simulink model "model"  (R2014a)
settings: Solver=ode45  StartTime=0.0  StopTime=10.0  MaxStep=1  MinStep=1  RelTol=1e-3
undefined symbols (not defined in the file or in its folder): a1, a2, a3, b1, b2, b3, H, T
settings Model: Creator=L13-4  LastModifiedBy=L13-4

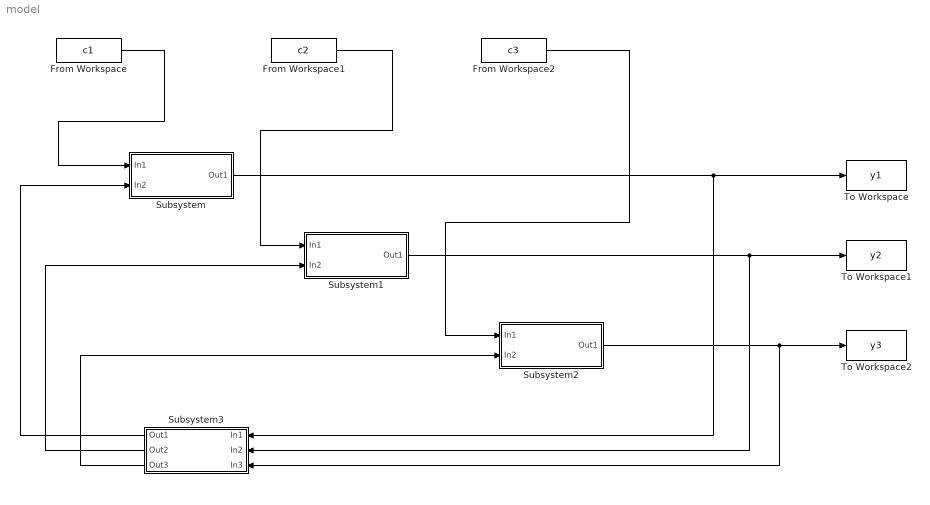
== system model ==
  From Workspace : FromWorkspace  VariableName=c1  SampleTime=0
  From Workspace1 : FromWorkspace  VariableName=c2  SampleTime=0
  From Workspace2 : FromWorkspace  VariableName=c3  SampleTime=0
  Subsystem : Subsystem
  Subsystem1 : Subsystem
  Subsystem2 : Subsystem
  Subsystem3 : Subsystem
  To Workspace : ToWorkspace  VariableName=y1  SampleTime=-1
  To Workspace1 : ToWorkspace  VariableName=y2  SampleTime=-1
  To Workspace2 : ToWorkspace  VariableName=y3  SampleTime=-1
  wires:
  From Workspace/1 -> Subsystem/1(In1)
  Subsystem/1(Out1) -> Subsystem3/1(In1), To Workspace/1
  From Workspace1/1 -> Subsystem1/1(In1)
  From Workspace2/1 -> Subsystem2/1(In1)
  Subsystem1/1(Out1) -> Subsystem3/2(In2), To Workspace1/1
  Subsystem2/1(Out1) -> Subsystem3/3(In3), To Workspace2/1
  Subsystem3/1(Out1) -> Subsystem/2(In2)
  Subsystem3/2(Out2) -> Subsystem1/2(In2)
  Subsystem3/3(Out3) -> Subsystem2/2(In2)

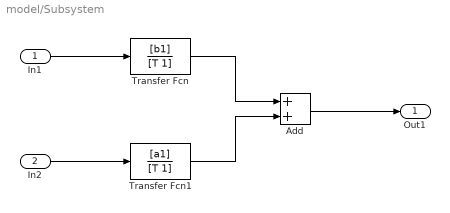
== system model/Subsystem ==
  In1 : Inport
  In2 : Inport  Port=2
  Add : Sum
  Transfer Fcn : TransferFcn  Numerator=[b1]  Denominator=[T 1]
  Transfer Fcn1 : TransferFcn  Numerator=[a1]  Denominator=[T 1]
  Out1 : Outport
  wires:
  In2/1 -> Transfer Fcn1/1
  Transfer Fcn1/1 -> Add/2
  Add/1 -> Out1/1
  Transfer Fcn/1 -> Add/1
  In1/1 -> Transfer Fcn/1

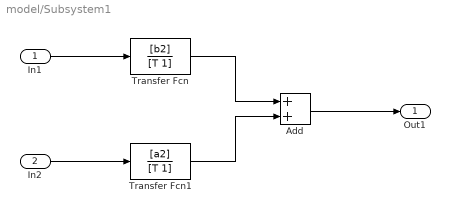
== system model/Subsystem1 ==
  In1 : Inport
  In2 : Inport  Port=2
  Add : Sum
  Transfer Fcn : TransferFcn  Numerator=[b2]  Denominator=[T 1]
  Transfer Fcn1 : TransferFcn  Numerator=[a2]  Denominator=[T 1]
  Out1 : Outport
  wires:
  In2/1 -> Transfer Fcn1/1
  Transfer Fcn1/1 -> Add/2
  Add/1 -> Out1/1
  Transfer Fcn/1 -> Add/1
  In1/1 -> Transfer Fcn/1

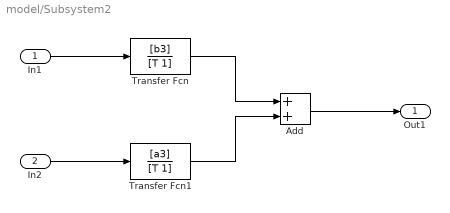
== system model/Subsystem2 ==
  In1 : Inport
  In2 : Inport  Port=2
  Add : Sum
  Transfer Fcn : TransferFcn  Numerator=[b3]  Denominator=[T 1]
  Transfer Fcn1 : TransferFcn  Numerator=[a3]  Denominator=[T 1]
  Out1 : Outport
  wires:
  In2/1 -> Transfer Fcn1/1
  Transfer Fcn1/1 -> Add/2
  Add/1 -> Out1/1
  Transfer Fcn/1 -> Add/1
  In1/1 -> Transfer Fcn/1

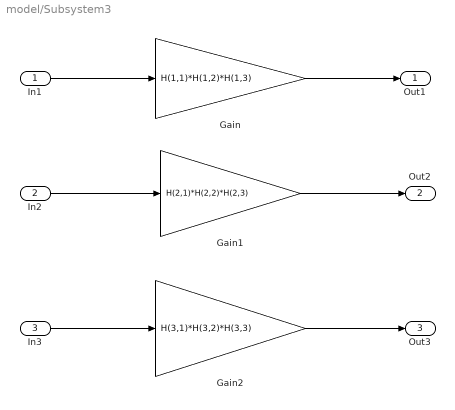
== system model/Subsystem3 ==
  In1 : Inport
  In2 : Inport  Port=2
  In3 : Inport  Port=3
  Gain : Gain  Gain=H(1,1)*H(1,2)*H(1,3)
  Gain1 : Gain  Gain=H(2,1)*H(2,2)*H(2,3)
  Gain2 : Gain  Gain=H(3,1)*H(3,2)*H(3,3)
  Out1 : Outport
  Out2 : Outport  Port=2
  Out3 : Outport  Port=3
  wires:
  In2/1 -> Gain1/1
  In1/1 -> Gain/1
  Gain/1 -> Out1/1
  Gain1/1 -> Out2/1
  In3/1 -> Gain2/1
  Gain2/1 -> Out3/1
